simulink model "PMSM_Model1"  (R2015b)
settings: Solver=VariableStepAuto  StartTime=0.0  StopTime=10.0  RelTol=1e-3
undefined symbols (not defined in the file): Lambda_f, Lambda_sd_0, Lambda_sq_0, Ls, p, Rs
settings Model: Creator=mihai.ciobanu  LastModifiedBy=mihai.ciobanu

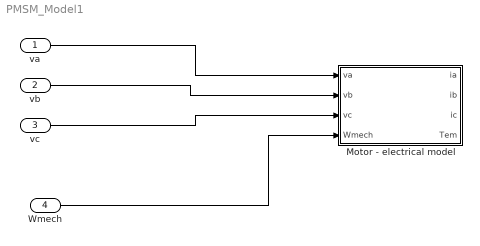
== system PMSM_Model1 ==
  va : Inport
  vb : Inport  Port=2
  vc : Inport  Port=3
  Wmech : Inport  Port=4
  Motor - electrical model : Subsystem
  wires:
  va/1 -> Motor - electrical model/1(va)
  vb/1 -> Motor - electrical model/2(vb)
  vc/1 -> Motor - electrical model/3(vc)
  Wmech/1 -> Motor - electrical model/4(Wmech)

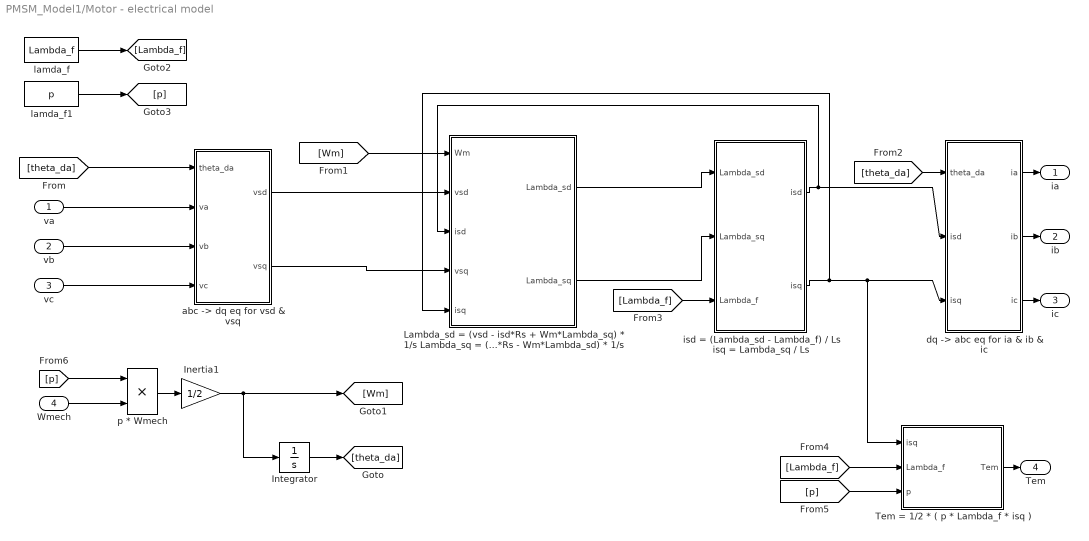
== system PMSM_Model1/Motor - electrical model ==
  va : Inport
  vb : Inport  Port=2
  vc : Inport  Port=3
  Wmech : Inport  Port=4
  Inertia1 : Gain  Gain=1/2  SaturateOnIntegerOverflow=on  OutDataTypeStr=Inherit: Same as input  ParamDataTypeStr=Inherit: Same as input
  Integrator : Integrator  InitialCondition=-pi/2
  Lambda_sd = (vsd - isd*Rs + Wm*Lambda_sq) * 1/s Lambda_sq = (vsd - isq*Rs - Wm*Lambda_sd) * 1/s : Subsystem
  Tem = 1/2 * ( p * Lambda_f * isq ) : Subsystem
  "abc -> dq eq for vsd & vsq" : Subsystem
  "dq -> abc eq for ia & ib & ic" : Subsystem
  isd = (Lambda_sd - Lambda_f) / Ls isq = Lambda_sq / Ls : Subsystem
  lamda_f : Constant  Value=Lambda_f  VectorParams1D=off
  lamda_f1 : Constant  Value=p  VectorParams1D=off
  p * Wmech : Product
  ia : Outport
  ib : Outport  Port=2
  ic : Outport  Port=3
  Tem : Outport  Port=4
  wires:
  Integrator/1 -> [theta_da]
  vb/1 -> "abc -> dq eq for vsd & vsq"/3(vb)
  vc/1 -> "abc -> dq eq for vsd & vsq"/4(vc)
  va/1 -> "abc -> dq eq for vsd & vsq"/2(va)
  [Wm] -> Lambda_sd = (vsd - isd*Rs + Wm*Lambda_sq) * 1/s Lambda_sq = (vsd - isq*Rs - Wm*Lambda_sd) * 1/s/1(Wm)
  [theta_da] -> "abc -> dq eq for vsd & vsq"/1(theta_da)
  "abc -> dq eq for vsd & vsq"/2(vsq) -> Lambda_sd = (vsd - isd*Rs + Wm*Lambda_sq) * 1/s Lambda_sq = (vsd - isq*Rs - Wm*Lambda_sd) * 1/s/4(vsq)
  "abc -> dq eq for vsd & vsq"/1(vsd) -> Lambda_sd = (vsd - isd*Rs + Wm*Lambda_sq) * 1/s Lambda_sq = (vsd - isq*Rs - Wm*Lambda_sd) * 1/s/2(vsd)
  Lambda_sd = (vsd - isd*Rs + Wm*Lambda_sq) * 1/s Lambda_sq = (vsd - isq*Rs - Wm*Lambda_sd) * 1/s/1(Lambda_sd) -> isd = (Lambda_sd - Lambda_f) / Ls isq = Lambda_sq / Ls/1(Lambda_sd)
  Lambda_sd = (vsd - isd*Rs + Wm*Lambda_sq) * 1/s Lambda_sq = (vsd - isq*Rs - Wm*Lambda_sd) * 1/s/2(Lambda_sq) -> isd = (Lambda_sd - Lambda_f) / Ls isq = Lambda_sq / Ls/2(Lambda_sq)
  [Lambda_f] -> Tem = 1/2 * ( p * Lambda_f * isq )/2(Lambda_f)
  isd = (Lambda_sd - Lambda_f) / Ls isq = Lambda_sq / Ls/1(isd) -> "dq -> abc eq for ia & ib & ic"/2(isd), Lambda_sd = (vsd - isd*Rs + Wm*Lambda_sq) * 1/s Lambda_sq = (vsd - isq*Rs - Wm*Lambda_sd) * 1/s/3(isd)
  isd = (Lambda_sd - Lambda_f) / Ls isq = Lambda_sq / Ls/2(isq) -> Tem = 1/2 * ( p * Lambda_f * isq )/1(isq), "dq -> abc eq for ia & ib & ic"/3(isq), Lambda_sd = (vsd - isd*Rs + Wm*Lambda_sq) * 1/s Lambda_sq = (vsd - isq*Rs - Wm*Lambda_sd) * 1/s/5(isq)
  Tem = 1/2 * ( p * Lambda_f * isq )/1(Tem) -> Tem/1
  lamda_f1/1 -> [p]
  "dq -> abc eq for ia & ib & ic"/3(ic) -> ic/1
  "dq -> abc eq for ia & ib & ic"/1(ia) -> ia/1
  "dq -> abc eq for ia & ib & ic"/2(ib) -> ib/1
  [Lambda_f] -> isd = (Lambda_sd - Lambda_f) / Ls isq = Lambda_sq / Ls/3(Lambda_f)
  [theta_da] -> "dq -> abc eq for ia & ib & ic"/1(theta_da)
  lamda_f/1 -> [Lambda_f]
  [p] -> Tem = 1/2 * ( p * Lambda_f * isq )/3(p)
  [p] -> p * Wmech/1
  Wmech/1 -> p * Wmech/2
  p * Wmech/1 -> Inertia1/1
  Inertia1/1 -> Integrator/1, [Wm]

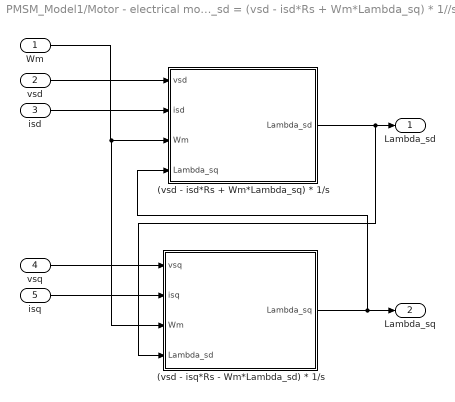
== system PMSM_Model1/Motor - electrical model/Lambda_sd = (vsd - isd*Rs + Wm*Lambda_sq) * 1//s Lambda_sq = (vsd - isq*Rs - Wm*Lambda_sd) * 1//s ==
  Wm : Inport
  vsd : Inport  Port=2
  isd : Inport  Port=3
  vsq : Inport  Port=4
  isq : Inport  Port=5
  (vsd - isd*Rs + Wm*Lambda_sq) * 1/s : Subsystem
  (vsd - isq*Rs - Wm*Lambda_sd) * 1/s : Subsystem
  Lambda_sd : Outport
  Lambda_sq : Outport  Port=2
  wires:
  (vsd - isq*Rs - Wm*Lambda_sd) * 1/s/1(Lambda_sq) -> (vsd - isd*Rs + Wm*Lambda_sq) * 1/s/4(Lambda_sq), Lambda_sq/1
  isd/1 -> (vsd - isd*Rs + Wm*Lambda_sq) * 1/s/2(isd)
  vsd/1 -> (vsd - isd*Rs + Wm*Lambda_sq) * 1/s/1(vsd)
  (vsd - isd*Rs + Wm*Lambda_sq) * 1/s/1(Lambda_sd) -> Lambda_sd/1, (vsd - isq*Rs - Wm*Lambda_sd) * 1/s/4(Lambda_sd)
  isq/1 -> (vsd - isq*Rs - Wm*Lambda_sd) * 1/s/2(isq)
  vsq/1 -> (vsd - isq*Rs - Wm*Lambda_sd) * 1/s/1(vsq)
  Wm/1 -> (vsd - isq*Rs - Wm*Lambda_sd) * 1/s/3(Wm), (vsd - isd*Rs + Wm*Lambda_sq) * 1/s/3(Wm)

== system PMSM_Model1/Motor - electrical model/Tem = 1//2 * ( p * Lambda_f * isq ) ==
  isq : Inport
  Lambda_f : Inport  Port=2
  p : Inport  Port=3
  Gain : Gain  Gain=1/2
  p * Lambda_f * isq : Product  Inputs=3
  Tem : Outport
  wires:
  p * Lambda_f * isq/1 -> Gain/1
  isq/1 -> p * Lambda_f * isq/1
  Lambda_f/1 -> p * Lambda_f * isq/2
  p/1 -> p * Lambda_f * isq/3
  Gain/1 -> Tem/1

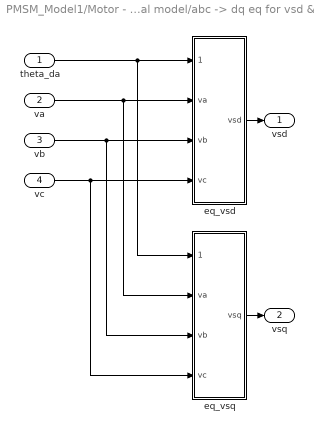
== system PMSM_Model1/Motor - electrical model/abc -> dq eq for vsd & vsq ==
  theta_da : Inport
  va : Inport  Port=2
  vb : Inport  Port=3
  vc : Inport  Port=4
  eq_vsd : Subsystem
  eq_vsq : Subsystem
  vsd : Outport
  vsq : Outport  Port=2
  wires:
  vb/1 -> eq_vsq/3(vb), eq_vsd/3(vb)
  vc/1 -> eq_vsq/4(vc), eq_vsd/4(vc)
  theta_da/1 -> eq_vsq/1(theta_da), eq_vsd/1(theta_da)
  va/1 -> eq_vsq/2(va), eq_vsd/2(va)
  eq_vsd/1(vsd) -> vsd/1
  eq_vsq/1(vsq) -> vsq/1

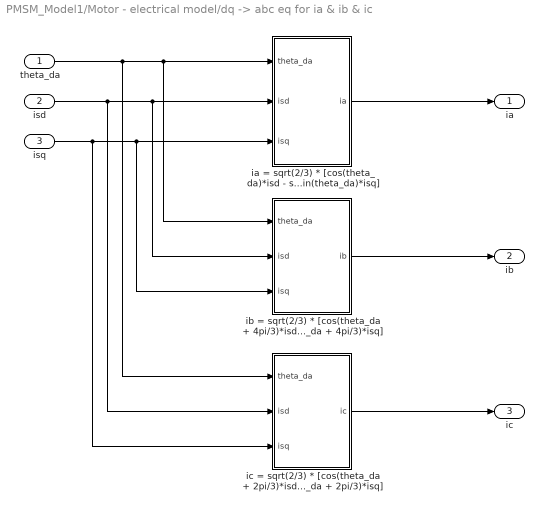
== system PMSM_Model1/Motor - electrical model/dq -> abc eq for ia & ib & ic ==
  theta_da : Inport
  isd : Inport  Port=2
  isq : Inport  Port=3
  ia = sqrt(2/3) * [cos(theta_da)*isd - sin(theta_da)*isq] : Subsystem
  ib = sqrt(2/3) * [cos(theta_da + 4pi/3)*isd - sin(theta_da + 4pi/3)*isq] : Subsystem
  ic = sqrt(2/3) * [cos(theta_da + 2pi/3)*isd - sin(theta_da + 2pi/3)*isq] : Subsystem
  ia : Outport
  ib : Outport  Port=2
  ic : Outport  Port=3
  wires:
  theta_da/1 -> ic = sqrt(2/3) * [cos(theta_da + 2pi/3)*isd - sin(theta_da + 2pi/3)*isq]/1(theta_da), ib = sqrt(2/3) * [cos(theta_da + 4pi/3)*isd - sin(theta_da + 4pi/3)*isq]/1(theta_da), ia = sqrt(2/3) * [cos(theta_da)*isd - sin(theta_da)*isq]/1(theta_da)
  isd/1 -> ic = sqrt(2/3) * [cos(theta_da + 2pi/3)*isd - sin(theta_da + 2pi/3)*isq]/2(isd), ib = sqrt(2/3) * [cos(theta_da + 4pi/3)*isd - sin(theta_da + 4pi/3)*isq]/2(isd), ia = sqrt(2/3) * [cos(theta_da)*isd - sin(theta_da)*isq]/2(isd)
  isq/1 -> ic = sqrt(2/3) * [cos(theta_da + 2pi/3)*isd - sin(theta_da + 2pi/3)*isq]/3(isq), ib = sqrt(2/3) * [cos(theta_da + 4pi/3)*isd - sin(theta_da + 4pi/3)*isq]/3(isq), ia = sqrt(2/3) * [cos(theta_da)*isd - sin(theta_da)*isq]/3(isq)
  ia = sqrt(2/3) * [cos(theta_da)*isd - sin(theta_da)*isq]/1(ia) -> ia/1
  ib = sqrt(2/3) * [cos(theta_da + 4pi/3)*isd - sin(theta_da + 4pi/3)*isq]/1(ib) -> ib/1
  ic = sqrt(2/3) * [cos(theta_da + 2pi/3)*isd - sin(theta_da + 2pi/3)*isq]/1(ic) -> ic/1

== system PMSM_Model1/Motor - electrical model/isd = (Lambda_sd - Lambda_f) // Ls isq = Lambda_sq // Ls ==
  Lambda_sd : Inport
  Lambda_sq : Inport  Port=2
  Lambda_f : Inport  Port=3
  (Lambda_sd - Lambda_f) / Ls : Subsystem
  Lambda_sq / Ls : Subsystem
  isd : Outport
  isq : Outport  Port=2
  wires:
  Lambda_sq/1 -> Lambda_sq / Ls/1(Lambda_sq)
  Lambda_sq / Ls/1(isq) -> isq/1
  Lambda_sd/1 -> (Lambda_sd - Lambda_f) / Ls/1(Lambda_sd)
  (Lambda_sd - Lambda_f) / Ls/1(isd) -> isd/1
  Lambda_f/1 -> (Lambda_sd - Lambda_f) / Ls/2(Lambda_f)

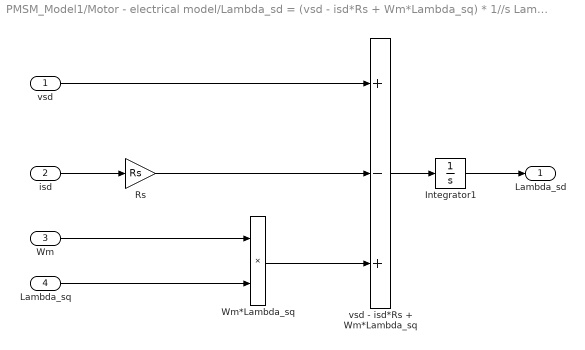
== system PMSM_Model1/Motor - electrical model/Lambda_sd = (vsd - isd*Rs + Wm*Lambda_sq) * 1//s Lambda_sq = (vsd - isq*Rs - Wm*Lambda_sd) * 1//s/(vsd - isd*Rs + Wm*Lambda_sq) * 1//s ==
  vsd : Inport
  isd : Inport  Port=2
  Wm : Inport  Port=3
  Lambda_sq : Inport  Port=4
  Integrator1 : Integrator  InitialCondition=[Lambda_sd_0; Lambda_sq_0]
  Rs : Gain  Gain=Rs
  Wm*Lambda_sq : Product
  vsd - isd*Rs + Wm*Lambda_sq : Sum  Inputs=+-+
  Lambda_sd : Outport
  wires:
  Lambda_sq/1 -> Wm*Lambda_sq/2
  Wm*Lambda_sq/1 -> vsd - isd*Rs + Wm*Lambda_sq/3
  isd/1 -> Rs/1
  Wm/1 -> Wm*Lambda_sq/1
  vsd/1 -> vsd - isd*Rs + Wm*Lambda_sq/1
  Rs/1 -> vsd - isd*Rs + Wm*Lambda_sq/2
  Integrator1/1 -> Lambda_sd/1
  vsd - isd*Rs + Wm*Lambda_sq/1 -> Integrator1/1

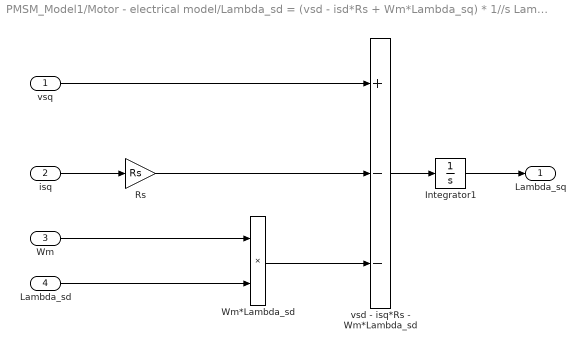
== system PMSM_Model1/Motor - electrical model/Lambda_sd = (vsd - isd*Rs + Wm*Lambda_sq) * 1//s Lambda_sq = (vsd - isq*Rs - Wm*Lambda_sd) * 1//s/(vsd - isq*Rs - Wm*Lambda_sd) * 1//s ==
  vsq : Inport
  isq : Inport  Port=2
  Wm : Inport  Port=3
  Lambda_sd : Inport  Port=4
  Integrator1 : Integrator  InitialCondition=[Lambda_sd_0; Lambda_sq_0]
  Rs : Gain  Gain=Rs
  Wm*Lambda_sd : Product
  vsd - isq*Rs - Wm*Lambda_sd : Sum  Inputs=+--
  Lambda_sq : Outport
  wires:
  Lambda_sd/1 -> Wm*Lambda_sd/2
  Wm*Lambda_sd/1 -> vsd - isq*Rs - Wm*Lambda_sd/3
  isq/1 -> Rs/1
  Wm/1 -> Wm*Lambda_sd/1
  vsq/1 -> vsd - isq*Rs - Wm*Lambda_sd/1
  Rs/1 -> vsd - isq*Rs - Wm*Lambda_sd/2
  Integrator1/1 -> Lambda_sq/1
  vsd - isq*Rs - Wm*Lambda_sd/1 -> Integrator1/1

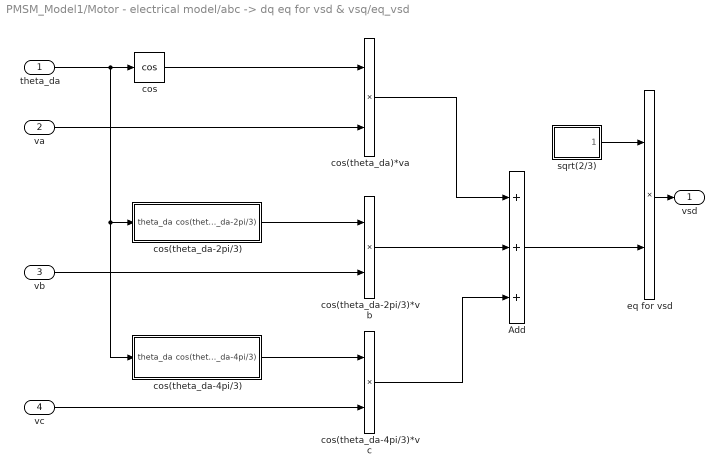
== system PMSM_Model1/Motor - electrical model/abc -> dq eq for vsd & vsq/eq_vsd ==
  theta_da : Inport
  va : Inport  Port=2
  vb : Inport  Port=3
  vc : Inport  Port=4
  Add : Sum  Inputs=+++
  cos : Trigonometry  Operator=cos
  cos(theta_da)*va : Product
  cos(theta_da-2pi/3) : Subsystem
  cos(theta_da-2pi/3)*vb : Product
  cos(theta_da-4pi/3) : Subsystem
  cos(theta_da-4pi/3)*vc : Product
  eq for vsd : Product
  sqrt(2/3) : Subsystem
  vsd : Outport
  wires:
  theta_da/1 -> cos(theta_da-4pi/3)/1(theta_da), cos(theta_da-2pi/3)/1(theta_da), cos/1
  vc/1 -> cos(theta_da-4pi/3)*vc/2
  cos(theta_da-2pi/3)/1(cos(theta_da-2pi/3)) -> cos(theta_da-2pi/3)*vb/1
  cos/1 -> cos(theta_da)*va/1
  cos(theta_da-4pi/3)/1(cos(theta_da-4pi/3)) -> cos(theta_da-4pi/3)*vc/1
  cos(theta_da-2pi/3)*vb/1 -> Add/2
  va/1 -> cos(theta_da)*va/2
  sqrt(2/3)/1(sqrt(2/3)) -> eq for vsd/1
  cos(theta_da-4pi/3)*vc/1 -> Add/3
  cos(theta_da)*va/1 -> Add/1
  vb/1 -> cos(theta_da-2pi/3)*vb/2
  eq for vsd/1 -> vsd/1
  Add/1 -> eq for vsd/2

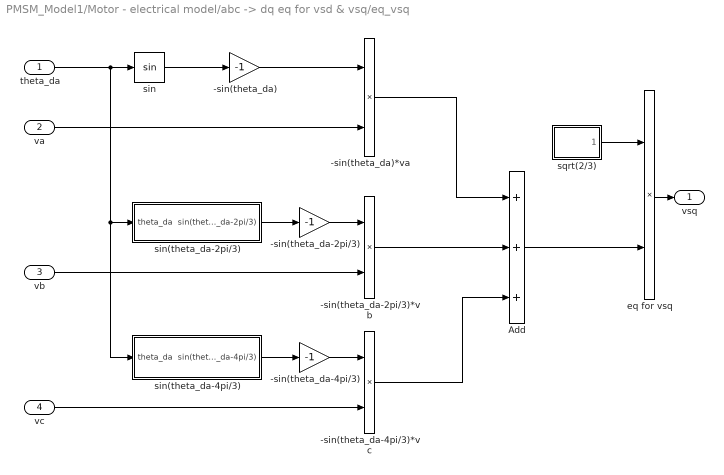
== system PMSM_Model1/Motor - electrical model/abc -> dq eq for vsd & vsq/eq_vsq ==
  theta_da : Inport
  va : Inport  Port=2
  vb : Inport  Port=3
  vc : Inport  Port=4
  -sin(theta_da) : Gain  Gain=-1
  -sin(theta_da)*va : Product
  -sin(theta_da-2pi/3) : Gain  Gain=-1
  -sin(theta_da-2pi/3)*vb : Product
  -sin(theta_da-4pi/3) : Gain  Gain=-1
  -sin(theta_da-4pi/3)*vc : Product
  Add : Sum  Inputs=+++
  eq for vsq : Product
  sin : Trigonometry
  sin(theta_da-2pi/3) : Subsystem
  sin(theta_da-4pi/3) : Subsystem
  sqrt(2/3) : Subsystem
  vsq : Outport
  wires:
  theta_da/1 -> sin(theta_da-4pi/3)/1(theta_da), sin(theta_da-2pi/3)/1(theta_da), sin/1
  vc/1 -> -sin(theta_da-4pi/3)*vc/2
  sin(theta_da-2pi/3)/1(sin(theta_da-2pi/3)) -> -sin(theta_da-2pi/3)/1
  sin/1 -> -sin(theta_da)/1
  sin(theta_da-4pi/3)/1(sin(theta_da-4pi/3)) -> -sin(theta_da-4pi/3)/1
  -sin(theta_da-2pi/3)*vb/1 -> Add/2
  va/1 -> -sin(theta_da)*va/2
  sqrt(2/3)/1(sqrt(2/3)) -> eq for vsq/1
  -sin(theta_da-4pi/3)*vc/1 -> Add/3
  -sin(theta_da)*va/1 -> Add/1
  vb/1 -> -sin(theta_da-2pi/3)*vb/2
  eq for vsq/1 -> vsq/1
  Add/1 -> eq for vsq/2
  -sin(theta_da)/1 -> -sin(theta_da)*va/1
  -sin(theta_da-2pi/3)/1 -> -sin(theta_da-2pi/3)*vb/1
  -sin(theta_da-4pi/3)/1 -> -sin(theta_da-4pi/3)*vc/1

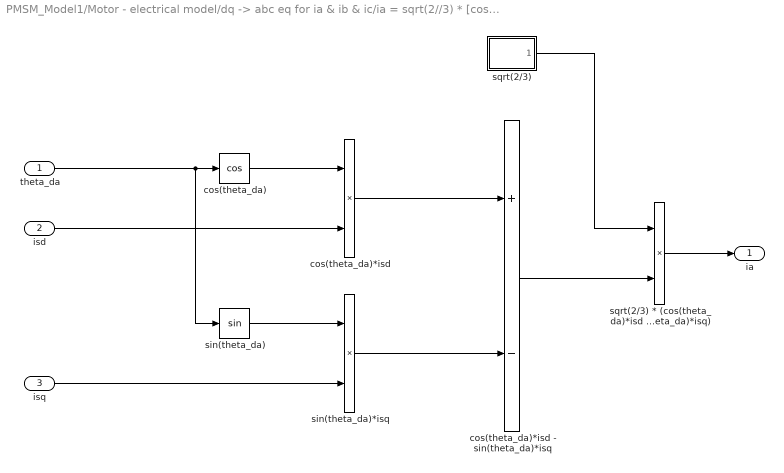
== system PMSM_Model1/Motor - electrical model/dq -> abc eq for ia & ib & ic/ia = sqrt(2//3) * [cos(theta_da)*isd - sin(theta_da)*isq] ==
  theta_da : Inport
  isd : Inport  Port=2
  isq : Inport  Port=3
  cos(theta_da) : Trigonometry  Operator=cos
  cos(theta_da)*isd : Product
  cos(theta_da)*isd - sin(theta_da)*isq : Sum  Inputs=+-
  sin(theta_da) : Trigonometry
  sin(theta_da)*isq : Product
  sqrt(2/3) : Subsystem
  sqrt(2/3) * (cos(theta_da)*isd - sin(theta_da)*isq) : Product
  ia : Outport
  wires:
  sqrt(2/3) * (cos(theta_da)*isd - sin(theta_da)*isq)/1 -> ia/1
  sin(theta_da)*isq/1 -> cos(theta_da)*isd - sin(theta_da)*isq/2
  isq/1 -> sin(theta_da)*isq/2
  sqrt(2/3)/1(sqrt(2/3)) -> sqrt(2/3) * (cos(theta_da)*isd - sin(theta_da)*isq)/1
  cos(theta_da)/1 -> cos(theta_da)*isd/1
  sin(theta_da)/1 -> sin(theta_da)*isq/1
  cos(theta_da)*isd/1 -> cos(theta_da)*isd - sin(theta_da)*isq/1
  cos(theta_da)*isd - sin(theta_da)*isq/1 -> sqrt(2/3) * (cos(theta_da)*isd - sin(theta_da)*isq)/2
  theta_da/1 -> sin(theta_da)/1, cos(theta_da)/1
  isd/1 -> cos(theta_da)*isd/2

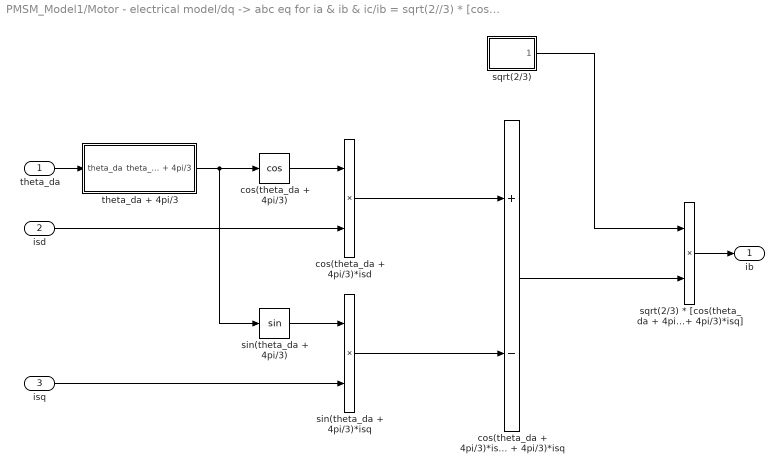
== system PMSM_Model1/Motor - electrical model/dq -> abc eq for ia & ib & ic/ib = sqrt(2//3) * [cos(theta_da + 4pi//3)*isd - sin(theta_da + 4pi//3)*isq] ==
  theta_da : Inport
  isd : Inport  Port=2
  isq : Inport  Port=3
  cos(theta_da + 4pi/3) : Trigonometry  Operator=cos
  cos(theta_da + 4pi/3)*isd : Product
  cos(theta_da + 4pi/3)*isd - sin(theta_da + 4pi/3)*isq : Sum  Inputs=+-
  sin(theta_da + 4pi/3) : Trigonometry
  sin(theta_da + 4pi/3)*isq : Product
  sqrt(2/3) : Subsystem
  sqrt(2/3) * [cos(theta_da + 4pi/3)*isd - sin(theta_da + 4pi/3)*isq] : Product
  theta_da + 4pi/3 : Subsystem
  ib : Outport
  wires:
  sqrt(2/3) * [cos(theta_da + 4pi/3)*isd - sin(theta_da + 4pi/3)*isq]/1 -> ib/1
  sin(theta_da + 4pi/3)*isq/1 -> cos(theta_da + 4pi/3)*isd - sin(theta_da + 4pi/3)*isq/2
  isq/1 -> sin(theta_da + 4pi/3)*isq/2
  sqrt(2/3)/1(sqrt(2/3)) -> sqrt(2/3) * [cos(theta_da + 4pi/3)*isd - sin(theta_da + 4pi/3)*isq]/1
  cos(theta_da + 4pi/3)/1 -> cos(theta_da + 4pi/3)*isd/1
  sin(theta_da + 4pi/3)/1 -> sin(theta_da + 4pi/3)*isq/1
  cos(theta_da + 4pi/3)*isd/1 -> cos(theta_da + 4pi/3)*isd - sin(theta_da + 4pi/3)*isq/1
  cos(theta_da + 4pi/3)*isd - sin(theta_da + 4pi/3)*isq/1 -> sqrt(2/3) * [cos(theta_da + 4pi/3)*isd - sin(theta_da + 4pi/3)*isq]/2
  isd/1 -> cos(theta_da + 4pi/3)*isd/2
  theta_da/1 -> theta_da + 4pi/3/1(theta_da)
  theta_da + 4pi/3/1(theta_da + 4pi/3) -> sin(theta_da + 4pi/3)/1, cos(theta_da + 4pi/3)/1

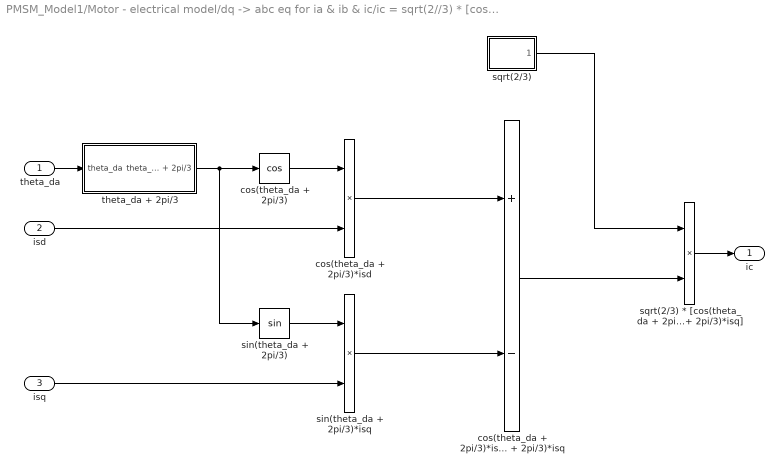
== system PMSM_Model1/Motor - electrical model/dq -> abc eq for ia & ib & ic/ic = sqrt(2//3) * [cos(theta_da + 2pi//3)*isd - sin(theta_da + 2pi//3)*isq] ==
  theta_da : Inport
  isd : Inport  Port=2
  isq : Inport  Port=3
  cos(theta_da + 2pi/3) : Trigonometry  Operator=cos
  cos(theta_da + 2pi/3)*isd : Product
  cos(theta_da + 2pi/3)*isd - sin(theta_da + 2pi/3)*isq : Sum  Inputs=+-
  sin(theta_da + 2pi/3) : Trigonometry
  sin(theta_da + 2pi/3)*isq : Product
  sqrt(2/3) : Subsystem
  sqrt(2/3) * [cos(theta_da + 2pi/3)*isd - sin(theta_da + 2pi/3)*isq] : Product
  theta_da + 2pi/3 : Subsystem
  ic : Outport
  wires:
  sqrt(2/3) * [cos(theta_da + 2pi/3)*isd - sin(theta_da + 2pi/3)*isq]/1 -> ic/1
  sin(theta_da + 2pi/3)*isq/1 -> cos(theta_da + 2pi/3)*isd - sin(theta_da + 2pi/3)*isq/2
  isq/1 -> sin(theta_da + 2pi/3)*isq/2
  sqrt(2/3)/1(sqrt(2/3)) -> sqrt(2/3) * [cos(theta_da + 2pi/3)*isd - sin(theta_da + 2pi/3)*isq]/1
  cos(theta_da + 2pi/3)/1 -> cos(theta_da + 2pi/3)*isd/1
  sin(theta_da + 2pi/3)/1 -> sin(theta_da + 2pi/3)*isq/1
  cos(theta_da + 2pi/3)*isd/1 -> cos(theta_da + 2pi/3)*isd - sin(theta_da + 2pi/3)*isq/1
  cos(theta_da + 2pi/3)*isd - sin(theta_da + 2pi/3)*isq/1 -> sqrt(2/3) * [cos(theta_da + 2pi/3)*isd - sin(theta_da + 2pi/3)*isq]/2
  isd/1 -> cos(theta_da + 2pi/3)*isd/2
  theta_da/1 -> theta_da + 2pi/3/1(theta_da)
  theta_da + 2pi/3/1(theta_da + 2pi/3) -> sin(theta_da + 2pi/3)/1, cos(theta_da + 2pi/3)/1

== system PMSM_Model1/Motor - electrical model/isd = (Lambda_sd - Lambda_f) // Ls isq = Lambda_sq // Ls/(Lambda_sd - Lambda_f) // Ls ==
  Lambda_sd : Inport
  Lambda_f : Inport  Port=2
  Gain : Gain  Gain=1/Ls
  Lambda_sd - Lambda_f : Sum  Inputs=+-
  isd : Outport
  wires:
  Lambda_f/1 -> Lambda_sd - Lambda_f/2
  Lambda_sd - Lambda_f/1 -> Gain/1
  Lambda_sd/1 -> Lambda_sd - Lambda_f/1
  Gain/1 -> isd/1

== system PMSM_Model1/Motor - electrical model/isd = (Lambda_sd - Lambda_f) // Ls isq = Lambda_sq // Ls/Lambda_sq // Ls ==
  Lambda_sq : Inport
  Gain : Gain  Gain=1/Ls
  isq : Outport
  wires:
  Lambda_sq/1 -> Gain/1
  Gain/1 -> isq/1

== system PMSM_Model1/Motor - electrical model/abc -> dq eq for vsd & vsq/eq_vsd/cos(theta_da-2pi//3) ==
  theta_da : Inport
  cos : Trigonometry  Operator=cos
  theta_da - 2pi/3 : Subsystem
  cos(theta_da-2pi/3) : Outport
  wires:
  theta_da/1 -> theta_da - 2pi/3/1(theta_da)
  cos/1 -> cos(theta_da-2pi/3)/1
  theta_da - 2pi/3/1(theta_da - 2pi/3) -> cos/1

== system PMSM_Model1/Motor - electrical model/abc -> dq eq for vsd & vsq/eq_vsd/cos(theta_da-4pi//3) ==
  theta_da : Inport
  cos : Trigonometry  Operator=cos
  theta_da - 4pi/3 : Subsystem
  cos(theta_da-4pi/3) : Outport
  wires:
  theta_da - 4pi/3/1(theta_da - 4pi/3) -> cos/1
  theta_da/1 -> theta_da - 4pi/3/1(theta_da)
  cos/1 -> cos(theta_da-4pi/3)/1

== system PMSM_Model1/Motor - electrical model/abc -> dq eq for vsd & vsq/eq_vsd/sqrt(2//3) ==
  2 : Constant  Value=2
  3 : Constant  Value=3
  Divide : Product  Inputs=*/
  Sqrt : Sqrt  SaturateOnIntegerOverflow=on
  sqrt(2/3) : Outport
  wires:
  Sqrt/1 -> sqrt(2/3)/1
  2/1 -> Divide/1
  3/1 -> Divide/2
  Divide/1 -> Sqrt/1

== system PMSM_Model1/Motor - electrical model/abc -> dq eq for vsd & vsq/eq_vsq/sin(theta_da-2pi//3) ==
  theta_da : Inport
  sin : Trigonometry
  theta_da - 2pi/3 : Subsystem
  sin(theta_da-2pi/3) : Outport
  wires:
  theta_da/1 -> theta_da - 2pi/3/1(theta_da)
  sin/1 -> sin(theta_da-2pi/3)/1
  theta_da - 2pi/3/1(theta_da - 2pi/3) -> sin/1

== system PMSM_Model1/Motor - electrical model/abc -> dq eq for vsd & vsq/eq_vsq/sin(theta_da-4pi//3) ==
  theta_da : Inport
  sin : Trigonometry
  theta_da - 4pi/3 : Subsystem
  sin(theta_da-4pi/3) : Outport
  wires:
  theta_da - 4pi/3/1(theta_da - 4pi/3) -> sin/1
  theta_da/1 -> theta_da - 4pi/3/1(theta_da)
  sin/1 -> sin(theta_da-4pi/3)/1

== system PMSM_Model1/Motor - electrical model/abc -> dq eq for vsd & vsq/eq_vsq/sqrt(2//3) ==
  2 : Constant  Value=2
  3 : Constant  Value=3
  Divide : Product  Inputs=*/
  Sqrt : Sqrt  SaturateOnIntegerOverflow=on
  sqrt(2/3) : Outport
  wires:
  Sqrt/1 -> sqrt(2/3)/1
  2/1 -> Divide/1
  3/1 -> Divide/2
  Divide/1 -> Sqrt/1

== system PMSM_Model1/Motor - electrical model/dq -> abc eq for ia & ib & ic/ia = sqrt(2//3) * [cos(theta_da)*isd - sin(theta_da)*isq]/sqrt(2//3) ==
  2 : Constant  Value=2
  3 : Constant  Value=3
  Divide : Product  Inputs=*/
  Sqrt : Sqrt  SaturateOnIntegerOverflow=on
  sqrt(2/3) : Outport
  wires:
  Sqrt/1 -> sqrt(2/3)/1
  2/1 -> Divide/1
  3/1 -> Divide/2
  Divide/1 -> Sqrt/1

== system PMSM_Model1/Motor - electrical model/dq -> abc eq for ia & ib & ic/ib = sqrt(2//3) * [cos(theta_da + 4pi//3)*isd - sin(theta_da + 4pi//3)*isq]/sqrt(2//3) ==
  2 : Constant  Value=2
  3 : Constant  Value=3
  Divide : Product  Inputs=*/
  Sqrt : Sqrt  SaturateOnIntegerOverflow=on
  sqrt(2/3) : Outport
  wires:
  Sqrt/1 -> sqrt(2/3)/1
  2/1 -> Divide/1
  3/1 -> Divide/2
  Divide/1 -> Sqrt/1

== system PMSM_Model1/Motor - electrical model/dq -> abc eq for ia & ib & ic/ib = sqrt(2//3) * [cos(theta_da + 4pi//3)*isd - sin(theta_da + 4pi//3)*isq]/theta_da + 4pi//3 ==
  theta_da : Inport
  4pi/3 : Subsystem
  Add : Sum
  theta_da + 4pi/3 : Outport
  wires:
  Add/1 -> theta_da + 4pi/3/1
  4pi/3/1(4pi/3) -> Add/2
  theta_da/1 -> Add/1

== system PMSM_Model1/Motor - electrical model/dq -> abc eq for ia & ib & ic/ic = sqrt(2//3) * [cos(theta_da + 2pi//3)*isd - sin(theta_da + 2pi//3)*isq]/sqrt(2//3) ==
  2 : Constant  Value=2
  3 : Constant  Value=3
  Divide : Product  Inputs=*/
  Sqrt : Sqrt  SaturateOnIntegerOverflow=on
  sqrt(2/3) : Outport
  wires:
  Sqrt/1 -> sqrt(2/3)/1
  2/1 -> Divide/1
  3/1 -> Divide/2
  Divide/1 -> Sqrt/1

== system PMSM_Model1/Motor - electrical model/dq -> abc eq for ia & ib & ic/ic = sqrt(2//3) * [cos(theta_da + 2pi//3)*isd - sin(theta_da + 2pi//3)*isq]/theta_da + 2pi//3 ==
  theta_da : Inport
  2pi/3 : Subsystem
  Add : Sum
  theta_da + 2pi/3 : Outport
  wires:
  Add/1 -> theta_da + 2pi/3/1
  2pi/3/1(2pi/3) -> Add/2
  theta_da/1 -> Add/1

== system PMSM_Model1/Motor - electrical model/abc -> dq eq for vsd & vsq/eq_vsd/cos(theta_da-2pi//3)/theta_da - 2pi//3 ==
  theta_da : Inport
  2pi/3 : Subsystem
  Add : Sum  Inputs=+-
  theta_da - 2pi/3 : Outport
  wires:
  Add/1 -> theta_da - 2pi/3/1
  2pi/3/1(2pi/3) -> Add/2
  theta_da/1 -> Add/1

== system PMSM_Model1/Motor - electrical model/abc -> dq eq for vsd & vsq/eq_vsd/cos(theta_da-4pi//3)/theta_da - 4pi//3 ==
  theta_da : Inport
  4pi/3 : Subsystem
  Add : Sum  Inputs=+-
  theta_da - 4pi/3 : Outport
  wires:
  Add/1 -> theta_da - 4pi/3/1
  4pi/3/1(4pi/3) -> Add/2
  theta_da/1 -> Add/1

== system PMSM_Model1/Motor - electrical model/abc -> dq eq for vsd & vsq/eq_vsq/sin(theta_da-2pi//3)/theta_da - 2pi//3 ==
  theta_da : Inport
  2pi/3 : Subsystem
  Add : Sum  Inputs=+-
  theta_da - 2pi/3 : Outport
  wires:
  Add/1 -> theta_da - 2pi/3/1
  2pi/3/1(2pi/3) -> Add/2
  theta_da/1 -> Add/1

== system PMSM_Model1/Motor - electrical model/abc -> dq eq for vsd & vsq/eq_vsq/sin(theta_da-4pi//3)/theta_da - 4pi//3 ==
  theta_da : Inport
  4pi/3 : Subsystem
  Add : Sum  Inputs=+-
  theta_da - 4pi/3 : Outport
  wires:
  Add/1 -> theta_da - 4pi/3/1
  4pi/3/1(4pi/3) -> Add/2
  theta_da/1 -> Add/1

== system PMSM_Model1/Motor - electrical model/dq -> abc eq for ia & ib & ic/ib = sqrt(2//3) * [cos(theta_da + 4pi//3)*isd - sin(theta_da + 4pi//3)*isq]/theta_da + 4pi//3/4pi//3 ==
  3 : Constant  Value=3
  4 : Constant  Value=4
  Divide : Product  Inputs=*/
  Product : Product
  pi : Constant  Value=pi
  4pi/3 : Outport
  wires:
  Product/1 -> Divide/1
  4/1 -> Product/1
  pi/1 -> Product/2
  3/1 -> Divide/2
  Divide/1 -> 4pi/3/1

== system PMSM_Model1/Motor - electrical model/dq -> abc eq for ia & ib & ic/ic = sqrt(2//3) * [cos(theta_da + 2pi//3)*isd - sin(theta_da + 2pi//3)*isq]/theta_da + 2pi//3/2pi//3 ==
  3 : Constant  Value=3
  4 : Constant  Value=2
  Divide : Product  Inputs=*/
  Product : Product
  pi : Constant  Value=pi
  2pi/3 : Outport
  wires:
  Product/1 -> Divide/1
  4/1 -> Product/1
  pi/1 -> Product/2
  3/1 -> Divide/2
  Divide/1 -> 2pi/3/1

== system PMSM_Model1/Motor - electrical model/abc -> dq eq for vsd & vsq/eq_vsd/cos(theta_da-2pi//3)/theta_da - 2pi//3/2pi//3 ==
  2 : Constant  Value=2
  3 : Constant  Value=3
  Divide : Product  Inputs=*/
  Product : Product
  pi : Constant  Value=pi
  2pi/3 : Outport
  wires:
  Product/1 -> Divide/1
  2/1 -> Product/1
  pi/1 -> Product/2
  3/1 -> Divide/2
  Divide/1 -> 2pi/3/1

== system PMSM_Model1/Motor - electrical model/abc -> dq eq for vsd & vsq/eq_vsd/cos(theta_da-4pi//3)/theta_da - 4pi//3/4pi//3 ==
  3 : Constant  Value=3
  4 : Constant  Value=4
  Divide : Product  Inputs=*/
  Product : Product
  pi : Constant  Value=pi
  4pi/3 : Outport
  wires:
  Product/1 -> Divide/1
  4/1 -> Product/1
  pi/1 -> Product/2
  3/1 -> Divide/2
  Divide/1 -> 4pi/3/1

== system PMSM_Model1/Motor - electrical model/abc -> dq eq for vsd & vsq/eq_vsq/sin(theta_da-2pi//3)/theta_da - 2pi//3/2pi//3 ==
  2 : Constant  Value=2
  3 : Constant  Value=3
  Divide : Product  Inputs=*/
  Product : Product
  pi : Constant  Value=pi
  2pi/3 : Outport
  wires:
  Product/1 -> Divide/1
  2/1 -> Product/1
  pi/1 -> Product/2
  3/1 -> Divide/2
  Divide/1 -> 2pi/3/1

== system PMSM_Model1/Motor - electrical model/abc -> dq eq for vsd & vsq/eq_vsq/sin(theta_da-4pi//3)/theta_da - 4pi//3/4pi//3 ==
  3 : Constant  Value=3
  4 : Constant  Value=4
  Divide : Product  Inputs=*/
  Product : Product
  pi : Constant  Value=pi
  4pi/3 : Outport
  wires:
  Product/1 -> Divide/1
  4/1 -> Product/1
  pi/1 -> Product/2
  3/1 -> Divide/2
  Divide/1 -> 4pi/3/1
